simulink model "Lab1_of_simulink_mohamed_faiad"  (R2021a)
settings: Solver=VariableStepAuto  StartTime=0.0  StopTime=10.0  RelTol=1e-3
settings Model: Creator=YasserNet  LastModifiedBy=YasserNet

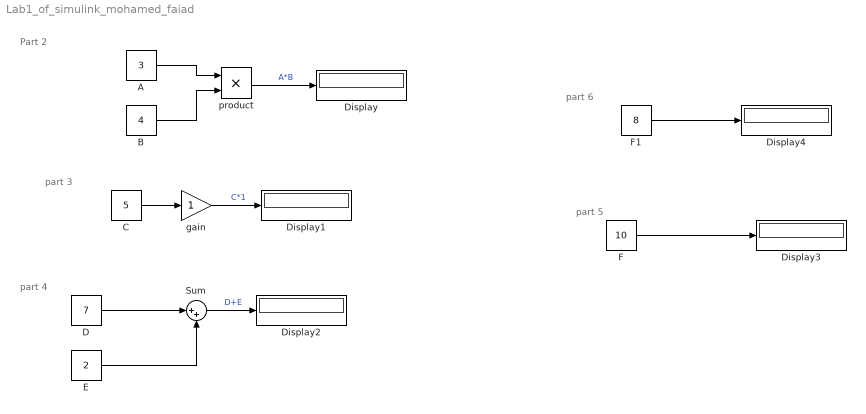
== system Lab1_of_simulink_mohamed_faiad ==
  note: part 6
  note: part 5
  note: part 4
  note: part 3
  note: Part 2
  A : Constant  Value=3
  B : Constant  Value=4
  C : Constant  Value=5
  D : Constant  Value=7
  Display{,1..4} (5 alike) : Display
  E : Constant  Value=2
  F : Constant  Value=10
  F1 : Constant  Value=8
  Sum : Sum  Inputs=|++
  gain : Gain
  product : Product
  wires:
  A/1 -> product/1
  B/1 -> product/2
  product/1 -> Display/1  "A*B"
  C/1 -> gain/1
  gain/1 -> Display1/1  "C*1"
  D/1 -> Sum/1
  E/1 -> Sum/2
  Sum/1 -> Display2/1  "D+E"
  F/1 -> Display3/1
  F1/1 -> Display4/1
